simulink model "Contactors"  (R2023b)
settings: Solver=FixedStepDiscrete  StartTime=0.0  StopTime=15  FixedStep=tSimCont  RelTol=1e-3
undefined symbols (not defined in the file): tSimCont
settings Model: DataDictionary=Contactors_data.sldd  Creator=Elio  LastModifiedBy=Elio

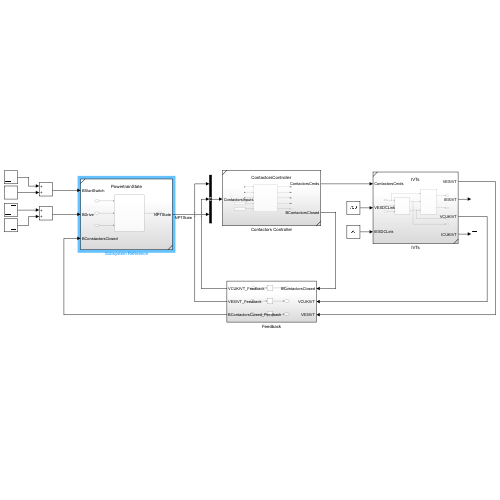
[thumbnail: Simulink's stored preview of the top-level diagram]
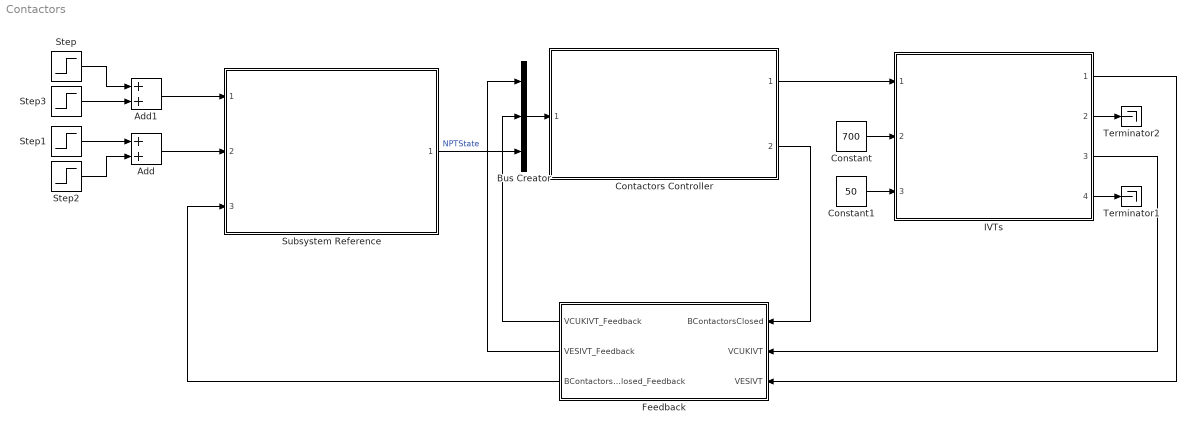
== system Contactors ==
  Add : Sum
  Add1 : Sum
  Bus Creator : BusCreator  Inputs=3  OutDataTypeStr=Bus: ContactorsInputs_BUS
      settings: InheritFromInputs=off
  Constant : Constant  Value=700  SampleTime=tSimCont
  Constant1 : Constant  Value=50  SampleTime=tSimCont
  Contactors Controller : Subsystem  ReferencedSubsystem=ContactorsController
      settings: PermitHierarchicalResolution=None
  Feedback : Subsystem
  IVTs : Subsystem  ReferencedSubsystem=IVTs
      settings: PermitHierarchicalResolution=None
  Step : Step  SampleTime=tSimCont
  Step1 : Step  Time=4  SampleTime=tSimCont
  Step2 : Step  Time=7  After=-1  SampleTime=tSimCont
  Step3 : Step  Time=10  After=-1  SampleTime=tSimCont
  Subsystem Reference : Subsystem  ReferencedSubsystem=PowertrainState
      settings: PermitHierarchicalResolution=None
  Terminator1 : Terminator
  Terminator2 : Terminator
  wires:
  Contactors Controller/1 -> IVTs/1
  Constant/1 -> IVTs/2
  Constant1/1 -> IVTs/3
  Contactors Controller/2 -> Feedback/1(BContactorsClosed)
  IVTs/1 -> Feedback/3(VESIVT)
  Bus Creator/1 -> Contactors Controller/1
  Feedback/2(VESIVT_Feedback) -> Bus Creator/1
  Feedback/1(VCUKIVT_Feedback) -> Bus Creator/2
  Subsystem Reference/1 -> Bus Creator/3  "NPTState"
  Feedback/3(BContactorsClosed_Feedback) -> Subsystem Reference/3
  IVTs/2 -> Terminator2/1
  IVTs/3 -> Feedback/2(VCUKIVT)
  IVTs/4 -> Terminator1/1
  Add/1 -> Subsystem Reference/2
  Step1/1 -> Add/1
  Step2/1 -> Add/2
  Add1/1 -> Subsystem Reference/1
  Step3/1 -> Add1/2
  Step/1 -> Add1/1

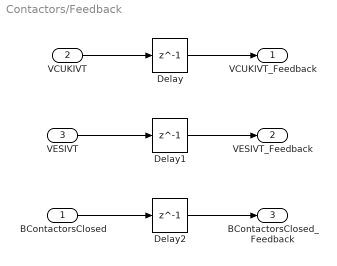
== system Contactors/Feedback ==
  BContactorsClosed : Inport
  VCUKIVT : Inport  Port=2
  VESIVT : Inport  Port=3
  Delay : Delay  DelayLength=1
  Delay1 : Delay  DelayLength=1
  Delay2 : Delay  DelayLength=1
  VCUKIVT_Feedback : Outport
  VESIVT_Feedback : Outport  Port=2
  BContactorsClosed_Feedback : Outport  Port=3
  wires:
  VCUKIVT/1 -> Delay/1
  Delay/1 -> VCUKIVT_Feedback/1
  VESIVT/1 -> Delay1/1
  Delay1/1 -> VESIVT_Feedback/1
  BContactorsClosed/1 -> Delay2/1
  Delay2/1 -> BContactorsClosed_Feedback/1
